simulink model "flexible_shafts"  (R2025a)
settings: Solver=VariableStepAuto  StartTime=0.0  StopTime=simlength  RelTol=1e-3
values from neighbouring files (symbols this model uses):
  K = lqr(A,B,Q,R)    [init_msmsm.m]
  simlength = 30    [init.m]    (also in init_msmsm.m)
  Tc = Ts    (= 0.001)    [init.m]    (also in init_msmsm.m)
libraries: nesl_utility x22, fl_lib x11, flexshaft_3masses_lib x2, flexshaft_lib x1
settings Model: Creator=dbagn  LastModifiedBy=dbagn
settings DataIOCC: SaveOutput=off  SignalLogging=off  DSMLogging=off  SaveTime=off  ReturnWorkspaceOutputs=off

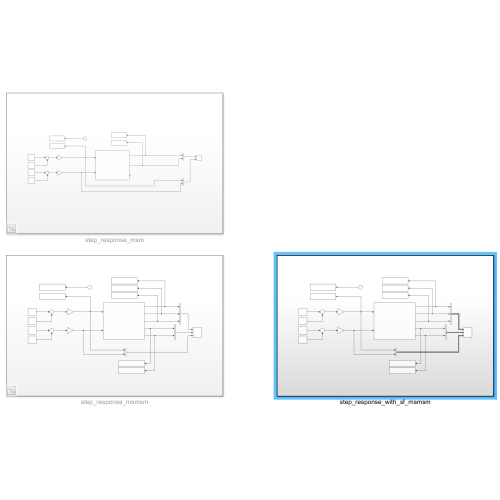
[thumbnail: Simulink's stored preview of the top-level diagram]
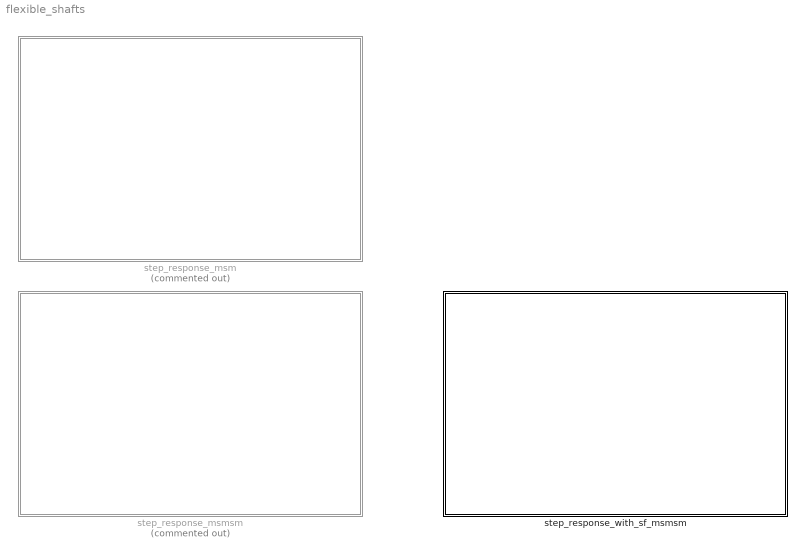
== system flexible_shafts ==
  step_response_msm : Subsystem  Commented=on
  step_response_msmsm : Subsystem  Commented=on
  step_response_with_sf_msmsm : Subsystem

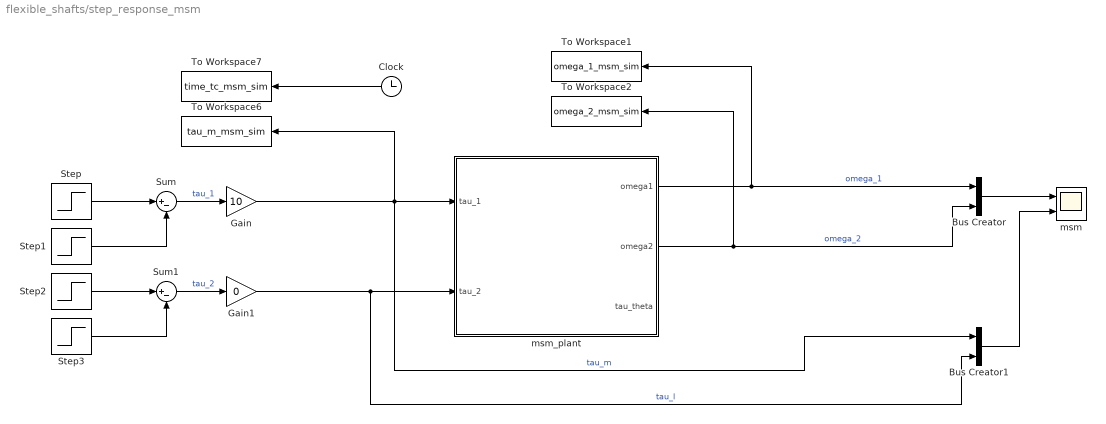
== system flexible_shafts/step_response_msm ==
  Bus Creator : BusCreator  Inputs=2
  Bus Creator1 : BusCreator  Inputs=2
  Clock : Clock
  Gain : Gain  Gain=10
  Gain1 : Gain  Gain=0
  Step : Step  Time=0.2  SampleTime=0
  Step1 : Step  Time=0.25  SampleTime=0
  Step2 : Step  Time=0.2+simlength/2  SampleTime=0
  Step3 : Step  Time=0.25+simlength/2  SampleTime=0
  Sum : Sum  Inputs=|+-
  Sum1 : Sum  Inputs=|+-
  To Workspace1 : ToWorkspace  VariableName=omega_1_msm_sim  SampleTime=Tc
      settings: MaxDataPoints=Nc
  To Workspace2 : ToWorkspace  VariableName=omega_2_msm_sim  SampleTime=Tc
      settings: MaxDataPoints=Nc
  To Workspace6 : ToWorkspace  VariableName=tau_m_msm_sim  SampleTime=Tc
      settings: MaxDataPoints=Nc
  To Workspace7 : ToWorkspace  VariableName=time_tc_msm_sim  SampleTime=Tc
      settings: MaxDataPoints=Nc
  msm : Scope  NumInputPorts=2
      settings: SampleTime=Tc  ActiveDisplayYMinimum=-0.50746122938016514  ActiveDisplayYMaximum=0.056384581042240554
  msm_plant : Subsystem
  wires:
  Step2/1 -> Sum1/1
  Sum1/1 -> Gain1/1  "tau_2"
  Step3/1 -> Sum1/2
  msm_plant/1(omega1) -> Bus Creator/1, To Workspace1/1  "omega_1"
  Clock/1 -> To Workspace7/1
  msm_plant/2(omega2) -> Bus Creator/2, To Workspace2/1  "omega_2"
  Sum/1 -> Gain/1  "tau_1"
  Step/1 -> Sum/1
  Step1/1 -> Sum/2
  Bus Creator1/1 -> msm/2
  Bus Creator/1 -> msm/1
  Gain/1 -> Bus Creator1/1, To Workspace6/1, msm_plant/1(tau_1)  "tau_m"
  Gain1/1 -> Bus Creator1/2, msm_plant/2(tau_2)  "tau_l"

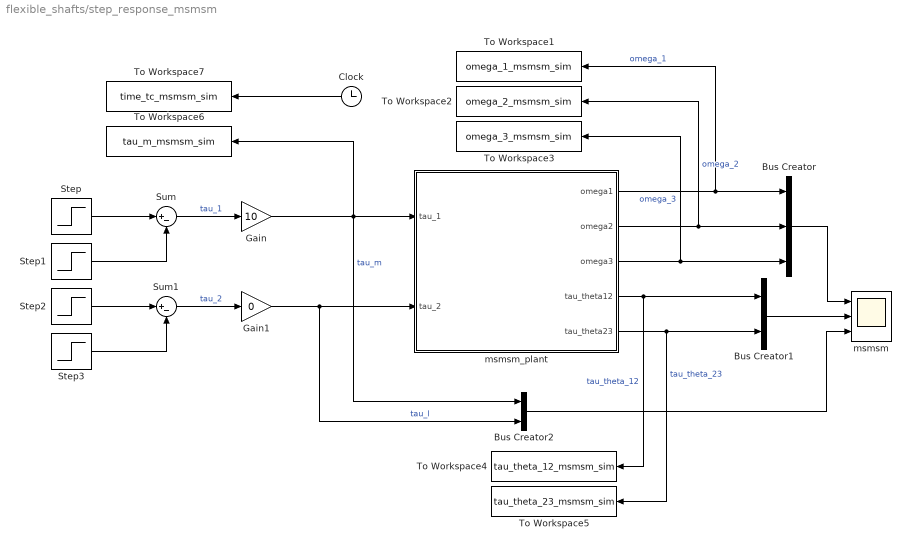
== system flexible_shafts/step_response_msmsm ==
  Bus Creator : BusCreator  Inputs=3
  Bus Creator1 : BusCreator  Inputs=2
  Bus Creator2 : BusCreator  Inputs=2
  Clock : Clock
  Gain : Gain  Gain=10
  Gain1 : Gain  Gain=0
  Step : Step  Time=0.2  SampleTime=0
  Step1 : Step  Time=0.25  SampleTime=0
  Step2 : Step  Time=0.2+simlength/2  SampleTime=0
  Step3 : Step  Time=0.25+simlength/2  SampleTime=0
  Sum : Sum  Inputs=|+-
  Sum1 : Sum  Inputs=|+-
  To Workspace1 : ToWorkspace  VariableName=omega_1_msmsm_sim  SampleTime=Tc
      settings: MaxDataPoints=Nc
  To Workspace2 : ToWorkspace  VariableName=omega_2_msmsm_sim  SampleTime=Tc
      settings: MaxDataPoints=Nc
  To Workspace3 : ToWorkspace  VariableName=omega_3_msmsm_sim  SampleTime=Tc
      settings: MaxDataPoints=Nc
  To Workspace4 : ToWorkspace  VariableName=tau_theta_12_msmsm_sim  SampleTime=Tc
      settings: MaxDataPoints=Nc
  To Workspace5 : ToWorkspace  VariableName=tau_theta_23_msmsm_sim  SampleTime=Tc
      settings: MaxDataPoints=Nc
  To Workspace6 : ToWorkspace  VariableName=tau_m_msmsm_sim  SampleTime=Tc
      settings: MaxDataPoints=Nc
  To Workspace7 : ToWorkspace  VariableName=time_tc_msmsm_sim  SampleTime=Tc
      settings: MaxDataPoints=Nc
  msmsm : Scope  NumInputPorts=3
      settings: SampleTime=Tc  ActiveDisplayYMinimum=-0.15054887911476209  ActiveDisplayYMaximum=0.54717891522703765
  msmsm_plant : Subsystem
  wires:
  Gain1/1 -> Bus Creator2/2, msmsm_plant/2(tau_2)  "tau_l"
  Step1/1 -> Sum/2
  Step/1 -> Sum/1
  Sum/1 -> Gain/1  "tau_1"
  Step3/1 -> Sum1/2
  Sum1/1 -> Gain1/1  "tau_2"
  Step2/1 -> Sum1/1
  msmsm_plant/3(omega3) -> To Workspace3/1, Bus Creator/3  "omega_3"
  Bus Creator/1 -> msmsm/1
  msmsm_plant/4(tau_theta12) -> To Workspace4/1, Bus Creator1/1  "tau_theta_12"
  msmsm_plant/5(tau_theta23) -> To Workspace5/1, Bus Creator1/2  "tau_theta_23"
  Bus Creator1/1 -> msmsm/2
  Bus Creator2/1 -> msmsm/3
  Gain/1 -> To Workspace6/1, Bus Creator2/1, msmsm_plant/1(tau_1)  "tau_m"
  msmsm_plant/2(omega2) -> Bus Creator/2, To Workspace2/1  "omega_2"
  Clock/1 -> To Workspace7/1
  msmsm_plant/1(omega1) -> Bus Creator/1, To Workspace1/1  "omega_1"

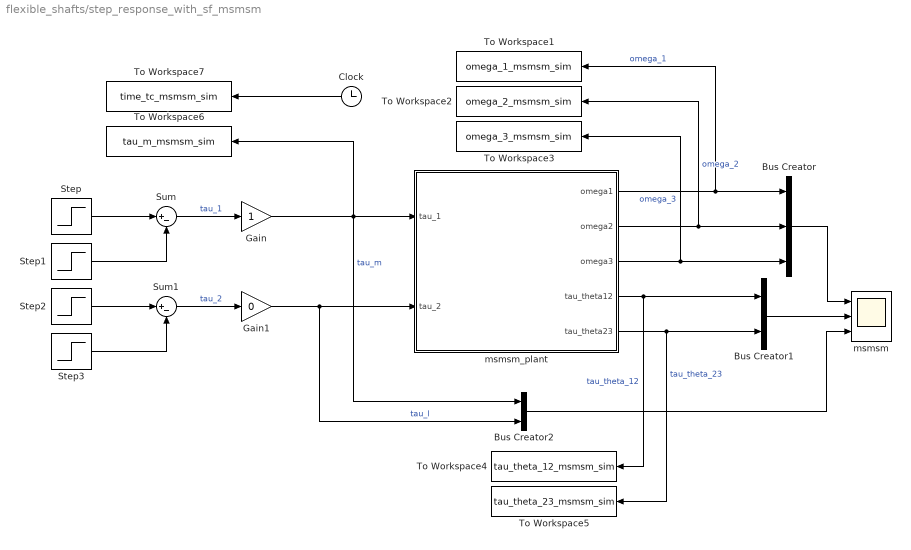
== system flexible_shafts/step_response_with_sf_msmsm ==
  Bus Creator : BusCreator  Inputs=3
  Bus Creator1 : BusCreator  Inputs=2
  Bus Creator2 : BusCreator  Inputs=2
  Clock : Clock
  Gain : Gain
  Gain1 : Gain  Gain=0
  Step : Step  Time=0.2  SampleTime=0
  Step1 : Step  Time=0.25  SampleTime=0
  Step2 : Step  Time=0.2+simlength/2  SampleTime=0
  Step3 : Step  Time=0.25+simlength/2  SampleTime=0
  Sum : Sum  Inputs=|+-
  Sum1 : Sum  Inputs=|+-
  To Workspace1 : ToWorkspace  VariableName=omega_1_msmsm_sim  SampleTime=Tc
      settings: MaxDataPoints=Nc
  To Workspace2 : ToWorkspace  VariableName=omega_2_msmsm_sim  SampleTime=Tc
      settings: MaxDataPoints=Nc
  To Workspace3 : ToWorkspace  VariableName=omega_3_msmsm_sim  SampleTime=Tc
      settings: MaxDataPoints=Nc
  To Workspace4 : ToWorkspace  VariableName=tau_theta_12_msmsm_sim  SampleTime=Tc
      settings: MaxDataPoints=Nc
  To Workspace5 : ToWorkspace  VariableName=tau_theta_23_msmsm_sim  SampleTime=Tc
      settings: MaxDataPoints=Nc
  To Workspace6 : ToWorkspace  VariableName=tau_m_msmsm_sim  SampleTime=Tc
      settings: MaxDataPoints=Nc
  To Workspace7 : ToWorkspace  VariableName=time_tc_msmsm_sim  SampleTime=Tc
      settings: MaxDataPoints=Nc
  msmsm : Scope  NumInputPorts=3
      settings: SampleTime=Tc  ActiveDisplayYMinimum=-0.70258693158847851  ActiveDisplayYMaximum=2.2617954056217231
  msmsm_plant : Subsystem
  wires:
  msmsm_plant/1(omega1) -> To Workspace1/1, Bus Creator/1  "omega_1"
  Clock/1 -> To Workspace7/1
  msmsm_plant/2(omega2) -> To Workspace2/1, Bus Creator/2  "omega_2"
  Gain/1 -> msmsm_plant/1(tau_1), Bus Creator2/1, To Workspace6/1  "tau_m"
  Bus Creator2/1 -> msmsm/3
  Bus Creator1/1 -> msmsm/2
  msmsm_plant/5(tau_theta23) -> Bus Creator1/2, To Workspace5/1  "tau_theta_23"
  msmsm_plant/4(tau_theta12) -> Bus Creator1/1, To Workspace4/1  "tau_theta_12"
  Bus Creator/1 -> msmsm/1
  msmsm_plant/3(omega3) -> Bus Creator/3, To Workspace3/1  "omega_3"
  Step2/1 -> Sum1/1
  Sum1/1 -> Gain1/1  "tau_2"
  Step3/1 -> Sum1/2
  Sum/1 -> Gain/1  "tau_1"
  Step/1 -> Sum/1
  Step1/1 -> Sum/2
  Gain1/1 -> msmsm_plant/2(tau_2), Bus Creator2/2  "tau_l"

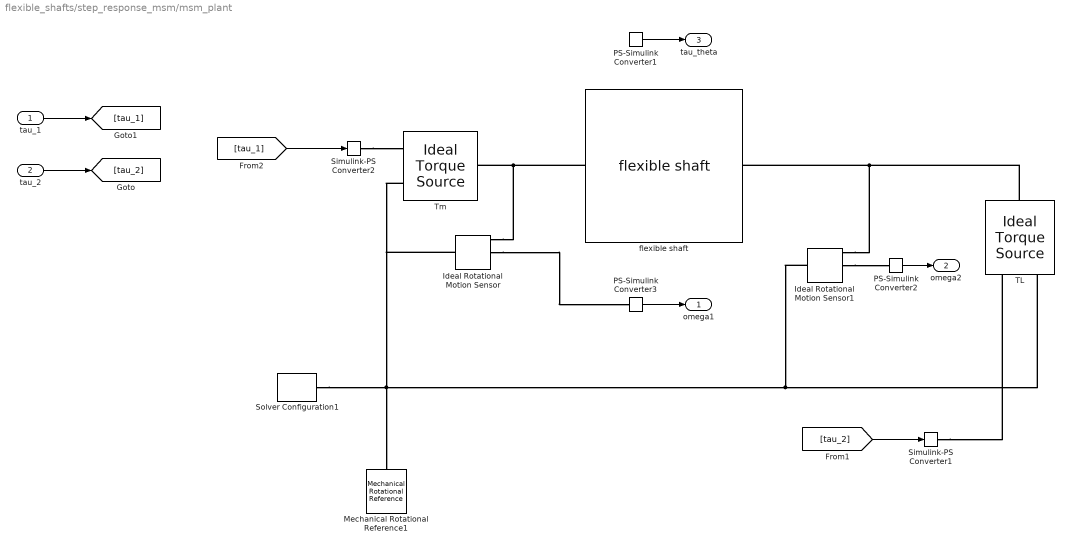
== system flexible_shafts/step_response_msm/msm_plant ==
  tau_1 : Inport
  tau_2 : Inport  Port=2
  Ideal Rotational Motion Sensor : fl_lib/Mechanical/Mechanical Sensors/Ideal Rotational Motion Sensor  reference=foundation.enum.MeasurementReference.difference  acceleration_port=false  velocity_port=true  position_port=true  wrap_angle=false  offset=0 rad
  Ideal Rotational Motion Sensor1 : fl_lib/Mechanical/Mechanical Sensors/Ideal Rotational Motion Sensor  reference=foundation.enum.MeasurementReference.difference  acceleration_port=false  velocity_port=true  position_port=true  wrap_angle=false  offset=0 rad
  Mechanical Rotational Reference1 : fl_lib/Mechanical/Rotational Elements/Mechanical Rotational Reference
  PS-Simulink Converter1 : nesl_utility/PS-Simulink Converter  PhysicalDomain=network_engine_domain  SubClassName=ps_output  LeftPortType=input  RightPortType=output  PseudoPeriodic=off  Frequencies=[]  VectorFormat=1-D array  Unit=1  AffineConversion=off
  PS-Simulink Converter2 : nesl_utility/PS-Simulink Converter  PhysicalDomain=network_engine_domain  SubClassName=ps_output  LeftPortType=input  RightPortType=output  PseudoPeriodic=off  Frequencies=[]  VectorFormat=1-D array  Unit=1  AffineConversion=off
  PS-Simulink Converter3 : nesl_utility/PS-Simulink Converter  PhysicalDomain=network_engine_domain  SubClassName=ps_output  LeftPortType=input  RightPortType=output  PseudoPeriodic=off  Frequencies=[]  VectorFormat=1-D array  Unit=1  AffineConversion=off
  Simulink-PS Converter1 : nesl_utility/Simulink-PS Converter  PhysicalDomain=network_engine_domain  SubClassName=ps_input  LeftPortType=input  RightPortType=output  PseudoPeriodic=off  Frequencies=[]  NoiseDistribution=none  NoiseParameters=[]  Unit=1  AffineConversion=off  FilteringAndDerivatives=provide  SimscapeFilterOrder=1  InputFilterTimeConstant=0.001  UdotUserProvided=0
  Simulink-PS Converter2 : nesl_utility/Simulink-PS Converter  PhysicalDomain=network_engine_domain  SubClassName=ps_input  LeftPortType=input  RightPortType=output  PseudoPeriodic=off  Frequencies=[]  NoiseDistribution=none  NoiseParameters=[]  Unit=1  AffineConversion=off  FilteringAndDerivatives=provide  SimscapeFilterOrder=1  InputFilterTimeConstant=0.001  UdotUserProvided=0
  Solver Configuration1 : nesl_utility/Solver Configuration  PhysicalDomain=network_engine_domain  SubClassName=solver  LeftPortType=input  RightPortType=generic  Tones=[]  Harmonics=[]  SimulateNoise=off  Profile=off  UseLocalSampling=off  EnableSwitchedLinearOptims=on  FrequencyDomain=off  UseCCode=off  RelTol=0.001  AbsTol=1e-06  MinStep=1e-09  ToWorkspace=off  RevertToSquareIcSolve=off  NumHomotopyIterations=100  PhasorMode=off  PhasorModeNumHarmonics=1  ConsistencySolver=NEWTON_FTOL  IndexReductionMethod=DerivativeReplacement  DoDC=off  ResidualTolerance=1e-09  ConsistencyTolSource=GLOBAL  ConsistencyAbsTol=0.001  ConsistencyRelTol=0.001  ConsistencyTolFactor=0.001  UseLocalSolver=off  LocalSolverChoice=NE_BACKWARD_EULER_ADVANCER  ResolveIndetEquations=on  FunctionEvalNumThread=1  LocalSolverSampleTime=0.001  DoFixedCost=off  MaxNonlinIter=3  MaxModeIter=2  ComputeImpulses=off  ImpulseIterations=2  LinearAlgebra=auto  LinearAlgebraNumThread=0  EquationFormulation=NE_TIME_EF  DelaysMemoryBudget=1024  AutomaticFiltering=on  FilteringTimeConstant=0.001  PartitionStorageMethod=AS_NEEDED  PartitionMemoryBudget=1024  PartitionMethod=ROBUST  MultibodyUseLocalSolver=off  MultibodyLocalSolverChoice=ODE1  MultibodyLocalSolverSampleTime=0.001
  TL : fl_lib/Mechanical/Mechanical Sources/Ideal Torque Source
  "Tm " : fl_lib/Mechanical/Mechanical Sources/Ideal Torque Source
  flexible shaft : flexshaft_lib/flexible shaft  b1=b1 N*m*s/rad  J1=J1 kg*m^2  b2=b2 N*m*s/rad  J2=J2 kg*m^2  b_theta=b_theta N*m*s/rad  k_theta=k_theta N*m/rad  w_1_specify=off  w_1_priority=None  w_1=0 rad/s  w_1_nominal_specify=off  w_1_nominal_value=1  w_1_nominal_unit=rad/s  w_2_specify=off  w_2_priority=None  w_2=0 rad/s  w_2_nominal_specify=off  w_2_nominal_value=1  w_2_nominal_unit=rad/s  t_1_specify=off  t_1_priority=None  t_1=0 N*m  t_1_nominal_specify=off  t_1_nominal_value=1  t_1_nominal_unit=N*m  t_2_specify=off  t_2_priority=None  t_2=0 N*m  t_2_nominal_specify=off  t_2_nominal_value=1  t_2_nominal_unit=N*m  t_theta_specify=off  t_theta_priority=None  t_theta=0 N*m  t_theta_nominal_specify=off  t_theta_nominal_value=1  t_theta_nominal_unit=N*m
      settings: InternalSimscapePortConfiguration="{\"Bottom\":[],\"Left\":[{\"id\":\"S1\",\"label\":\"S1\",\"type\":\"foundation.mechanical.rotational.rotational\"}],\"Right\":[{\"id\":\"S2\",\"label\":\"S2\",\"type\":\"foundation.mechanical.rotational.rotational\"}],\"Top\":[]}"
  omega1 : Outport
  omega2 : Outport  Port=2
  tau_theta : Outport  Port=3
  wires:
  PS-Simulink Converter3/1 -> omega1/1
  PS-Simulink Converter2/1 -> omega2/1
  tau_1/1 -> [tau_1]
  tau_2/1 -> [tau_2]
  [tau_1] -> Simulink-PS Converter2/1
  [tau_2] -> Simulink-PS Converter1/1
  PS-Simulink Converter1/1 -> tau_theta/1
  connections:
  Simulink-PS Converter2/RConn1 -- "Tm "/RConn1
  flexible shaft/LConn1 -- Ideal Rotational Motion Sensor/RConn1 -- "Tm "/LConn1
  Simulink-PS Converter1/RConn1 -- TL/RConn1
  TL/LConn1 -- flexible shaft/RConn1 -- Ideal Rotational Motion Sensor1/RConn1
  Solver Configuration1/RConn1 -- Ideal Rotational Motion Sensor/LConn1 -- "Tm "/RConn2 -- Mechanical Rotational Reference1/LConn1 -- Ideal Rotational Motion Sensor1/LConn1 -- TL/RConn2
  Ideal Rotational Motion Sensor/RConn2 -- PS-Simulink Converter3/LConn1
  Ideal Rotational Motion Sensor1/RConn2 -- PS-Simulink Converter2/LConn1

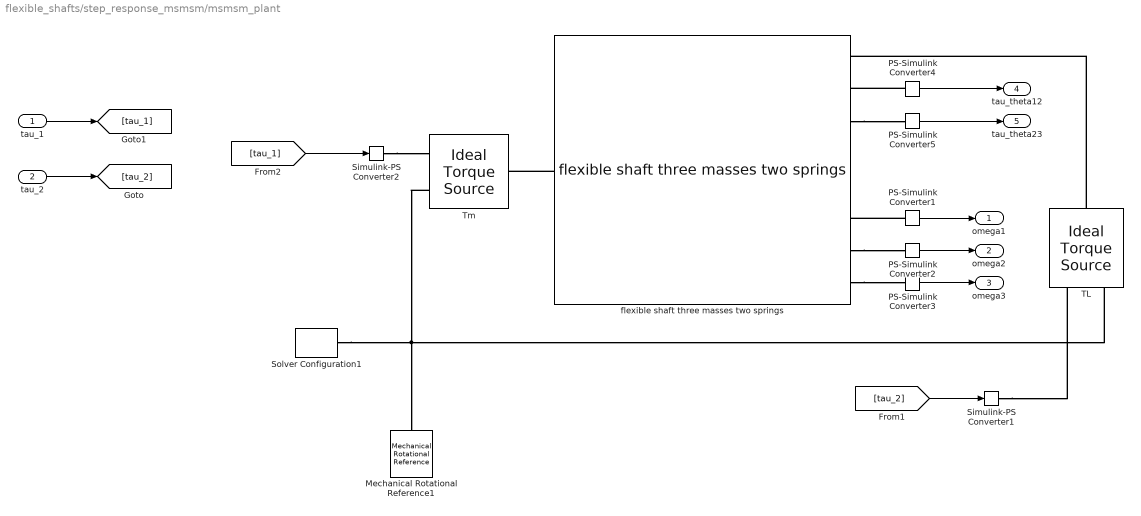
== system flexible_shafts/step_response_msmsm/msmsm_plant ==
  tau_1 : Inport
  tau_2 : Inport  Port=2
  Mechanical Rotational Reference1 : fl_lib/Mechanical/Rotational Elements/Mechanical Rotational Reference
  PS-Simulink Converter{1..5} (5 alike) : nesl_utility/PS-Simulink Converter  PhysicalDomain=network_engine_domain  SubClassName=ps_output  LeftPortType=input  RightPortType=output  PseudoPeriodic=off  Frequencies=[]  VectorFormat=1-D array  Unit=1  AffineConversion=off
  Simulink-PS Converter1 : nesl_utility/Simulink-PS Converter  PhysicalDomain=network_engine_domain  SubClassName=ps_input  LeftPortType=input  RightPortType=output  PseudoPeriodic=off  Frequencies=[]  NoiseDistribution=none  NoiseParameters=[]  Unit=1  AffineConversion=off  FilteringAndDerivatives=provide  SimscapeFilterOrder=1  InputFilterTimeConstant=0.001  UdotUserProvided=0
  Simulink-PS Converter2 : nesl_utility/Simulink-PS Converter  PhysicalDomain=network_engine_domain  SubClassName=ps_input  LeftPortType=input  RightPortType=output  PseudoPeriodic=off  Frequencies=[]  NoiseDistribution=none  NoiseParameters=[]  Unit=1  AffineConversion=off  FilteringAndDerivatives=provide  SimscapeFilterOrder=1  InputFilterTimeConstant=0.001  UdotUserProvided=0
  Solver Configuration1 : nesl_utility/Solver Configuration  PhysicalDomain=network_engine_domain  SubClassName=solver  LeftPortType=input  RightPortType=generic  Tones=[]  Harmonics=[]  SimulateNoise=off  Profile=off  UseLocalSampling=off  EnableSwitchedLinearOptims=on  FrequencyDomain=off  UseCCode=off  RelTol=0.001  AbsTol=1e-06  MinStep=1e-09  ToWorkspace=off  RevertToSquareIcSolve=off  NumHomotopyIterations=100  PhasorMode=off  PhasorModeNumHarmonics=1  ConsistencySolver=NEWTON_FTOL  IndexReductionMethod=DerivativeReplacement  DoDC=off  ResidualTolerance=1e-09  ConsistencyTolSource=GLOBAL  ConsistencyAbsTol=0.001  ConsistencyRelTol=0.001  ConsistencyTolFactor=0.001  UseLocalSolver=off  LocalSolverChoice=NE_BACKWARD_EULER_ADVANCER  ResolveIndetEquations=on  FunctionEvalNumThread=1  LocalSolverSampleTime=0.001  DoFixedCost=off  MaxNonlinIter=3  MaxModeIter=2  ComputeImpulses=off  ImpulseIterations=2  LinearAlgebra=auto  LinearAlgebraNumThread=0  EquationFormulation=NE_TIME_EF  DelaysMemoryBudget=1024  AutomaticFiltering=on  FilteringTimeConstant=0.001  PartitionStorageMethod=AS_NEEDED  PartitionMemoryBudget=1024  PartitionMethod=ROBUST  MultibodyUseLocalSolver=off  MultibodyLocalSolverChoice=ODE1  MultibodyLocalSolverSampleTime=0.001
  TL : fl_lib/Mechanical/Mechanical Sources/Ideal Torque Source
  "Tm " : fl_lib/Mechanical/Mechanical Sources/Ideal Torque Source
  flexible shaft three masses two springs : flexshaft_3masses_lib/flexible shaft three masses two springs  b1=b1 N*m*s/rad  J1=J1 kg*m^2  b2=b2 N*m*s/rad  J2=J2 kg*m^2  b3=b3 N*m*s/rad  J3=J3 kg*m^2  b_theta=b_theta N*m*s/rad  k_theta=k_theta N*m/rad  omega_1_specify=off  omega_1_priority=None  omega_1=0 rad/s  omega_1_nominal_specify=off  omega_1_nominal_value=1  omega_1_nominal_unit=rad/s  omega_2_specify=off  omega_2_priority=None  omega_2=0 rad/s  omega_2_nominal_specify=off  omega_2_nominal_value=1  omega_2_nominal_unit=rad/s  omega_3_specify=off  omega_3_priority=None  omega_3=0 rad/s  omega_3_nominal_specify=off  omega_3_nominal_value=1  omega_3_nominal_unit=rad/s  t_m_specify=off  t_m_priority=None  t_m=0 N*m  t_m_nominal_specify=off  t_m_nominal_value=1  t_m_nominal_unit=N*m  t_l_specify=off  t_l_priority=None  t_l=0 N*m  t_l_nominal_specify=off  t_l_nominal_value=1  t_l_nominal_unit=N*m  t_theta12_specify=off  t_theta12_priority=None  t_theta12=0 N*m  t_theta12_nominal_specify=off  t_theta12_nominal_value=1  t_theta12_nominal_unit=N*m  t_theta23_specify=off  t_theta23_priority=None  t_theta23=0 N*m  t_theta23_nominal_specify=off  t_theta23_nominal_value=1  t_theta23_nominal_unit=N*m
      settings: InternalSimscapePortConfiguration="{\"Bottom\":[],\"Left\":[{\"id\":\"Sm\",\"label\":\"Sm\",\"type\":\"foundation.mechanical.rotational.rotational\"}],\"Right\":[{\"id\":\"Sl\",\"label\":\"Sl\",\"type\":\"foundation.mechanical.rotational.rotational\"},{\"id\":\"tau_theta12\",\"label\":\"tau_theta12\",\"type\":\"output\"},{\"id\":\"tau_theta23\",\"label\":\"tau_theta23\",\"type\":\"output\"},{\"id\":\"tau_m\",\"label\":\"tau_m\",\"type\":\"output\"},{\"id\":\"tau_l\",\"label\":\"tau_l\",\"type\":\"output\"},{\"id\":\"omega1\",\"label\":\"omega1\",\"type\":\"output\"},{\"id\":\"omega2\",\"label\":\"omega2\",\"type\":\"output\"},{\"id\":\"omega3\",\"label\":\"omega3\",\"type\":\"output\"}],\"Top\":[]}"
  omega1 : Outport
  omega2 : Outport  Port=2
  omega3 : Outport  Port=3
  tau_theta12 : Outport  Port=4
  tau_theta23 : Outport  Port=5
  wires:
  [tau_2] -> Simulink-PS Converter1/1
  [tau_1] -> Simulink-PS Converter2/1
  tau_2/1 -> [tau_2]
  tau_1/1 -> [tau_1]
  PS-Simulink Converter4/1 -> tau_theta12/1
  PS-Simulink Converter5/1 -> tau_theta23/1
  PS-Simulink Converter2/1 -> omega2/1
  PS-Simulink Converter1/1 -> omega1/1
  PS-Simulink Converter3/1 -> omega3/1
  connections:
  TL/RConn2 -- Mechanical Rotational Reference1/LConn1 -- "Tm "/RConn2 -- Solver Configuration1/RConn1
  TL/LConn1 -- flexible shaft three masses two springs/RConn1
  Simulink-PS Converter1/RConn1 -- TL/RConn1
  flexible shaft three masses two springs/LConn1 -- "Tm "/LConn1
  Simulink-PS Converter2/RConn1 -- "Tm "/RConn1
  PS-Simulink Converter1/LConn1 -- flexible shaft three masses two springs/RConn6
  flexible shaft three masses two springs/RConn7 -- PS-Simulink Converter2/LConn1
  flexible shaft three masses two springs/RConn8 -- PS-Simulink Converter3/LConn1
  PS-Simulink Converter4/LConn1 -- flexible shaft three masses two springs/RConn2
  flexible shaft three masses two springs/RConn3 -- PS-Simulink Converter5/LConn1

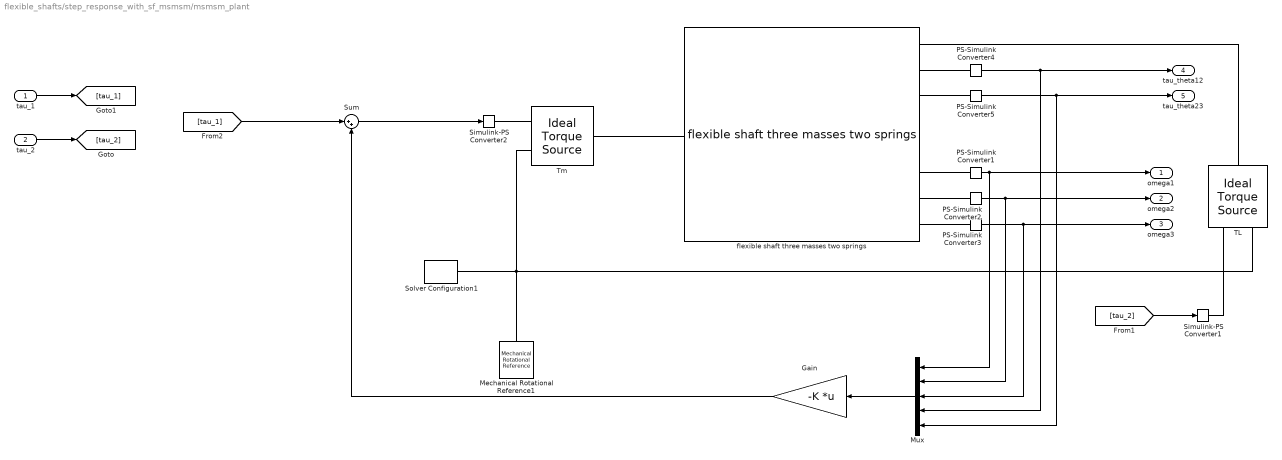
== system flexible_shafts/step_response_with_sf_msmsm/msmsm_plant ==
  tau_1 : Inport
  tau_2 : Inport  Port=2
  Gain : Gain  Gain=-K  Multiplication=Matrix(K*u)
  Mechanical Rotational Reference1 : fl_lib/Mechanical/Rotational Elements/Mechanical Rotational Reference
  Mux : Mux  Inputs=5
  PS-Simulink Converter{1..5} (5 alike) : nesl_utility/PS-Simulink Converter  PhysicalDomain=network_engine_domain  SubClassName=ps_output  LeftPortType=input  RightPortType=output  PseudoPeriodic=off  Frequencies=[]  VectorFormat=1-D array  Unit=1  AffineConversion=off
  Simulink-PS Converter1 : nesl_utility/Simulink-PS Converter  PhysicalDomain=network_engine_domain  SubClassName=ps_input  LeftPortType=input  RightPortType=output  PseudoPeriodic=off  Frequencies=[]  NoiseDistribution=none  NoiseParameters=[]  Unit=1  AffineConversion=off  FilteringAndDerivatives=provide  SimscapeFilterOrder=1  InputFilterTimeConstant=0.001  UdotUserProvided=0
  Simulink-PS Converter2 : nesl_utility/Simulink-PS Converter  PhysicalDomain=network_engine_domain  SubClassName=ps_input  LeftPortType=input  RightPortType=output  PseudoPeriodic=off  Frequencies=[]  NoiseDistribution=none  NoiseParameters=[]  Unit=1  AffineConversion=off  FilteringAndDerivatives=provide  SimscapeFilterOrder=1  InputFilterTimeConstant=0.001  UdotUserProvided=0
  Solver Configuration1 : nesl_utility/Solver Configuration  PhysicalDomain=network_engine_domain  SubClassName=solver  LeftPortType=input  RightPortType=generic  Tones=[]  Harmonics=[]  SimulateNoise=off  Profile=off  UseLocalSampling=off  EnableSwitchedLinearOptims=on  FrequencyDomain=off  UseCCode=off  RelTol=0.001  AbsTol=1e-06  MinStep=1e-09  ToWorkspace=off  RevertToSquareIcSolve=off  NumHomotopyIterations=100  PhasorMode=off  PhasorModeNumHarmonics=1  ConsistencySolver=NEWTON_FTOL  IndexReductionMethod=DerivativeReplacement  DoDC=off  ResidualTolerance=1e-09  ConsistencyTolSource=GLOBAL  ConsistencyAbsTol=0.001  ConsistencyRelTol=0.001  ConsistencyTolFactor=0.001  UseLocalSolver=off  LocalSolverChoice=NE_BACKWARD_EULER_ADVANCER  ResolveIndetEquations=on  FunctionEvalNumThread=1  LocalSolverSampleTime=0.001  DoFixedCost=off  MaxNonlinIter=3  MaxModeIter=2  ComputeImpulses=off  ImpulseIterations=2  LinearAlgebra=auto  LinearAlgebraNumThread=0  EquationFormulation=NE_TIME_EF  DelaysMemoryBudget=1024  AutomaticFiltering=on  FilteringTimeConstant=0.001  PartitionStorageMethod=AS_NEEDED  PartitionMemoryBudget=1024  PartitionMethod=ROBUST  MultibodyUseLocalSolver=off  MultibodyLocalSolverChoice=ODE1  MultibodyLocalSolverSampleTime=0.001
  Sum : Sum  Inputs=|++
  TL : fl_lib/Mechanical/Mechanical Sources/Ideal Torque Source
  "Tm " : fl_lib/Mechanical/Mechanical Sources/Ideal Torque Source
  flexible shaft three masses two springs : flexshaft_3masses_lib/flexible shaft three masses two springs  b1=b1 N*m*s/rad  J1=J1 kg*m^2  b2=b2 N*m*s/rad  J2=J2 kg*m^2  b3=b3 N*m*s/rad  J3=J3 kg*m^2  b_theta=b_theta N*m*s/rad  k_theta=k_theta N*m/rad  omega_1_specify=off  omega_1_priority=None  omega_1=0 rad/s  omega_1_nominal_specify=off  omega_1_nominal_value=1  omega_1_nominal_unit=rad/s  omega_2_specify=off  omega_2_priority=None  omega_2=0 rad/s  omega_2_nominal_specify=off  omega_2_nominal_value=1  omega_2_nominal_unit=rad/s  omega_3_specify=off  omega_3_priority=None  omega_3=0 rad/s  omega_3_nominal_specify=off  omega_3_nominal_value=1  omega_3_nominal_unit=rad/s  t_m_specify=off  t_m_priority=None  t_m=0 N*m  t_m_nominal_specify=off  t_m_nominal_value=1  t_m_nominal_unit=N*m  t_l_specify=off  t_l_priority=None  t_l=0 N*m  t_l_nominal_specify=off  t_l_nominal_value=1  t_l_nominal_unit=N*m  t_theta12_specify=off  t_theta12_priority=None  t_theta12=0 N*m  t_theta12_nominal_specify=off  t_theta12_nominal_value=1  t_theta12_nominal_unit=N*m  t_theta23_specify=off  t_theta23_priority=None  t_theta23=0 N*m  t_theta23_nominal_specify=off  t_theta23_nominal_value=1  t_theta23_nominal_unit=N*m
      settings: InternalSimscapePortConfiguration="{\"Bottom\":[],\"Left\":[{\"id\":\"Sm\",\"label\":\"Sm\",\"type\":\"foundation.mechanical.rotational.rotational\"}],\"Right\":[{\"id\":\"Sl\",\"label\":\"Sl\",\"type\":\"foundation.mechanical.rotational.rotational\"},{\"id\":\"tau_theta12\",\"label\":\"tau_theta12\",\"type\":\"output\"},{\"id\":\"tau_theta23\",\"label\":\"tau_theta23\",\"type\":\"output\"},{\"id\":\"tau_m\",\"label\":\"tau_m\",\"type\":\"output\"},{\"id\":\"tau_l\",\"label\":\"tau_l\",\"type\":\"output\"},{\"id\":\"omega1\",\"label\":\"omega1\",\"type\":\"output\"},{\"id\":\"omega2\",\"label\":\"omega2\",\"type\":\"output\"},{\"id\":\"omega3\",\"label\":\"omega3\",\"type\":\"output\"}],\"Top\":[]}"
  omega1 : Outport
  omega2 : Outport  Port=2
  omega3 : Outport  Port=3
  tau_theta12 : Outport  Port=4
  tau_theta23 : Outport  Port=5
  wires:
  PS-Simulink Converter3/1 -> Mux/3, omega3/1
  PS-Simulink Converter1/1 -> Mux/1, omega1/1
  PS-Simulink Converter2/1 -> Mux/2, omega2/1
  PS-Simulink Converter5/1 -> tau_theta23/1, Mux/5
  PS-Simulink Converter4/1 -> Mux/4, tau_theta12/1
  tau_1/1 -> [tau_1]
  tau_2/1 -> [tau_2]
  [tau_2] -> Simulink-PS Converter1/1
  Mux/1 -> Gain/1
  Sum/1 -> Simulink-PS Converter2/1
  [tau_1] -> Sum/1
  Gain/1 -> Sum/2
  connections:
  flexible shaft three masses two springs/RConn3 -- PS-Simulink Converter5/LConn1
  PS-Simulink Converter4/LConn1 -- flexible shaft three masses two springs/RConn2
  flexible shaft three masses two springs/RConn8 -- PS-Simulink Converter3/LConn1
  flexible shaft three masses two springs/RConn7 -- PS-Simulink Converter2/LConn1
  PS-Simulink Converter1/LConn1 -- flexible shaft three masses two springs/RConn6
  Simulink-PS Converter2/RConn1 -- "Tm "/RConn1
  flexible shaft three masses two springs/LConn1 -- "Tm "/LConn1
  Simulink-PS Converter1/RConn1 -- TL/RConn1
  TL/LConn1 -- flexible shaft three masses two springs/RConn1
  Solver Configuration1/RConn1 -- "Tm "/RConn2 -- Mechanical Rotational Reference1/LConn1 -- TL/RConn2
